simulink model "gm_sampleModel1941_sub"  (R2023a)
settings: Solver=VariableStepAuto  StartTime=0.0  StopTime=10.0  RelTol=1e-3
libraries: simulink x1, hdlsllib x1
settings Model: Creator=user1  LastModifiedBy=user1
settings OptimizationCC: BlockReduction=off  ConditionallyExecuteInputs=off
settings DebuggingCC: InheritedTsInSrcMsg=none

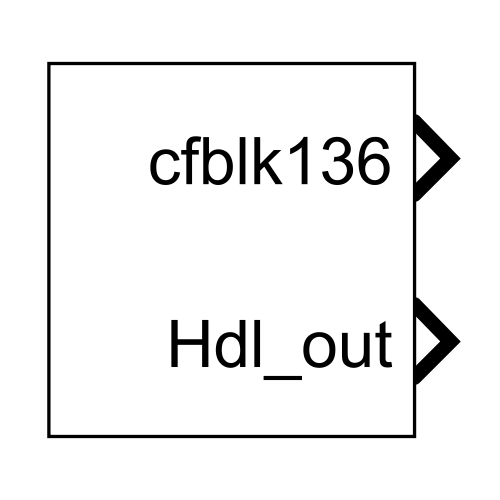
[thumbnail: Simulink's stored preview of the top-level diagram]
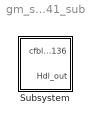
== system gm_sampleModel1941_sub ==
  Subsystem : Subsystem

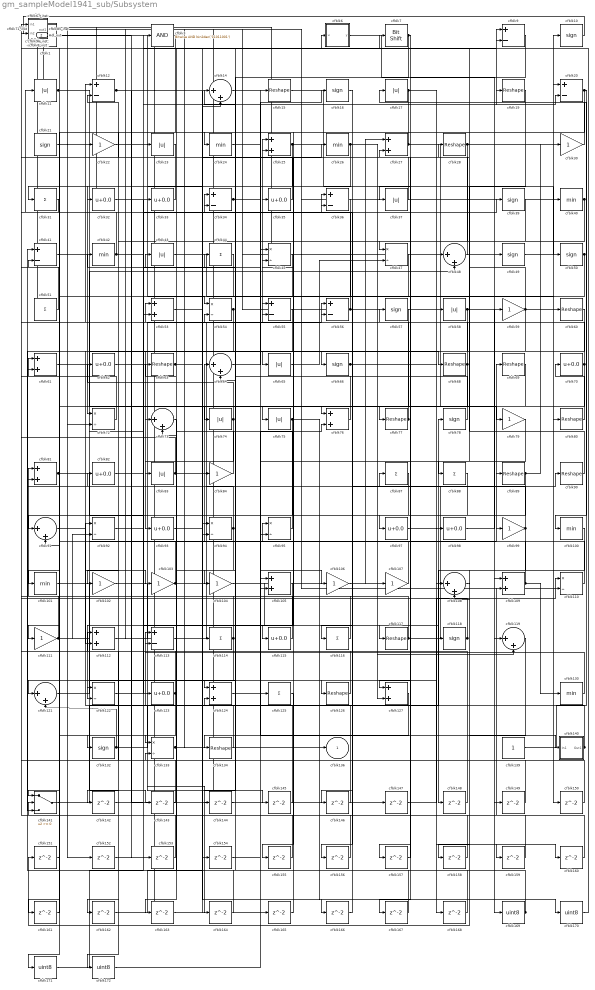
== system gm_sampleModel1941_sub/Subsystem ==
  cfblk1 : Subsystem  mask(Detect Rise Nonnegative){vinit=double(0), InputProcessing=Elements as channels (sample based), OutDataTypeStr=uint8}
      mask prompts: vinit "Simulink:masks:InitialCondition_MP"; InputProcessing "Simulink:masks:InputProcessing_MP"; OutDataTypeStr "Simulink:masks:OutputDataType_MP"
      mask help: Simulink:masks:DetectRiseNonnegative_MD
      mask init:
      | InputProcessing = 'Elements as channels (sample based)';
      | OutDataTypeStr = 'uint8';
      | vinit = double(0);
      mask TypeOptions InputProcessing: Simulink:masks:ColumnsAsChannelsFrameBased | Simulink:masks:ElementsAsChannelsSampleBased
      mask TypeOptions OutDataTypeStr: Simulink:masks:uint8 | Simulink:masks:boolean
      mask Display: fprintf('U >= 0\n&  NOT\nU/z >= 0')
  cfblk{10,16,21,39,49..50,57,66,78,118,132} (11 alike) : Signum
  cfblk{24,26,40,42,100..101,130} (7 alike) : MinMax  OutDataTypeStr=uint8
  cfblk{22,30,59,79,84,99,102..104,106..107,111} (12 alike) : Gain  OutDataTypeStr=uint8
  cfblk{25,27,53,61,76,81,105,109,112,124,127} (11 alike) : Sum  OutDataTypeStr=uint8
  cfblk{14,48,64,73,91,108,119,121} (8 alike) : Sum  Inputs=|++  OutDataTypeStr=uint8
  cfblk{11,17,23,37,43,58,65,74..75,83} (10 alike) : Abs  OutDataTypeStr=uint8  SaturateOnIntegerOverflow=off
  cfblk{45,47,54,72,92,94..95,110,122,133} (10 alike) : Product  Inputs=*/  OutDataTypeStr=uint8  RndMeth=Zero  SaturateOnIntegerOverflow=on
  cfblk{9,12,20,34,36,41,55..56,113} (9 alike) : Sum  Inputs=+-  OutDataTypeStr=uint8
  cfblk{31,44,51,87..88,114,116,125} (8 alike) : Sum  Inputs=+  OutDataTypeStr=uint8
  cfblk{32..33,35,62,70,82,93,97..98,115,123} (11 alike) : Bias  Bias=0.0  SaturateOnIntegerOverflow=off
  cfblk{15,19,28,60,63,68..69,77,80,89..90,117,126,134} (14 alike) : Reshape
  cfblk120_inst : Subsystem
  cfblk128_inst : Subsystem
  cfblk129_inst : Subsystem
  cfblk139 : Constant  OutDataTypeStr=uint8  SampleTime=-1
  cfblk13_inst : Subsystem
  cfblk140 : Subsystem
  cfblk141 : Switch  OutDataTypeStr=uint8  SaturateOnIntegerOverflow=off  InputSameDT=off
  cfblk{142..168} (27 alike) : Delay  SampleTime=1
  cfblk{169..172} (4 alike) : DataTypeConversion  OutDataTypeStr=uint8  SaturateOnIntegerOverflow=off  RndMeth=Floor
  cfblk18_inst : Subsystem
  cfblk2 : Constant  Value=0  OutDataTypeStr=uint8  SampleTime=1
  cfblk29_inst : Subsystem
  cfblk3 : simulink/Logic and Bit Operations/Bitwise Operator  logicop=AND  UseBitMask=on  BitMask=bin2dec('11011001')  BitMaskRealWorld=Stored Integer
      settings: LibrarySourceBlock=|
      | hdlsllib/Logic and Bit
      | Operations/Bitwise
      | Operator
  cfblk4 : Constant  Value=0  OutDataTypeStr=uint8  SampleTime=1
  cfblk46_inst : Subsystem
  cfblk5 : Constant  Value=0  OutDataTypeStr=uint8  SampleTime=1
  cfblk6 : Subsystem  mask(Compare To Constant){relop=<=, const=double(3), OutDataTypeStr=uint8, ZeroCross=on}
      mask prompts: relop "Simulink:masks:Operator_MP"; const "Simulink:masks:ConstantValue_MP"; OutDataTypeStr "Simulink:masks:OutputDataType_MP"; ZeroCross "Simulink:masks:EnableZerocrossingDetection_MP"
      mask help: Simulink:masks:CompareToConstant_MD
      mask init:
      | OutDataTypeStr = 'uint8';
      | ZeroCross = 'on';
      | blkName = 'sampleModel1941_sub/Subsystem/cfblk6';
      | const = double(3);
      | const_str = '3.0';
      | const_val = double(3);
      | relop = '<=';
      | setValue = 'fixdt(0, 8)';
      | str = '<= 3';
      mask TypeOptions relop: == | ~= | < | <= | >= | >
      mask TypeOptions OutDataTypeStr: Simulink:masks:uint8 | Simulink:masks:boolean
      mask Callback ZeroCross: sl('zeroCrossEnable', gcbh);
      mask Display: disp(str)
  cfblk67_inst : Subsystem
  cfblk7 : hdlsllib/Logic and Bit Operations/Bit Shift  mode=Shift Left Logical  N=0
  cfblk71_inst : Subsystem
  cfblk85_inst : Subsystem
  cfblk8_inst : Subsystem
  cfblk96_inst : Subsystem
  cfblk136 : Outport  OutDataTypeStr=uint8  SampleTime=1  VectorParamsAs1DForOutWhenUnconnected=off
  Hdl_out : Outport  Port=2  OutDataTypeStr=uint8  SampleTime=1
  wires:
  cfblk1/1(Y) -> cfblk54/1
  cfblk10/1 -> cfblk128_inst/2(in2)
  cfblk100/1 -> cfblk148/1
  cfblk101/1 -> cfblk143/1
  cfblk102/1 -> cfblk164/1
  cfblk103/1 -> cfblk41/2, cfblk25/1
  cfblk104/1 -> cfblk117/1
  cfblk105/1 -> cfblk122/2
  cfblk106/1 -> cfblk27/1
  cfblk107/1 -> cfblk46_inst/2(in2)
  cfblk108/1 -> cfblk151/1
  cfblk109/1 -> cfblk69/1, cfblk130/1
  cfblk11/1 -> cfblk75/1, Hdl_out/1
  cfblk110/1 -> cfblk35/1
  cfblk111/1 -> cfblk67_inst/2(in2), cfblk48/2, cfblk92/2, cfblk168/1
  cfblk112/1 -> cfblk56/1
  cfblk113/1 -> cfblk89/1
  cfblk114/1 -> cfblk8_inst/2(in2), cfblk121/1
  cfblk115/1 -> cfblk81/1
  cfblk116/1 -> cfblk61/1
  cfblk117/1 -> cfblk90/1, cfblk55/1
  cfblk118/1 -> cfblk71_inst/1(in1), cfblk120_inst/1(in1)
  cfblk119/1 -> cfblk158/1
  cfblk12/1 -> cfblk154/1, cfblk153/1
  cfblk120_inst/1(out1) -> cfblk21/1, cfblk107/1
  cfblk121/1 -> cfblk64/1
  cfblk122/1 -> cfblk145/1
  cfblk123/1 -> cfblk67_inst/1(in1), cfblk161/1
  cfblk124/1 -> cfblk125/1
  cfblk125/1 -> cfblk155/1
  cfblk126/1 -> cfblk46_inst/1(in1)
  cfblk127/1 -> cfblk134/1
  cfblk128_inst/1(out1) -> cfblk15/1
  cfblk129_inst/1(out1) -> cfblk96_inst/2(in2), cfblk152/1, cfblk136/1
  cfblk13_inst/1(out1) -> cfblk50/1
  cfblk130/1 -> cfblk113/1
  cfblk132/1 -> cfblk124/2, cfblk121/2
  cfblk133/1 -> cfblk99/1, cfblk166/1
  cfblk134/1 -> cfblk113/2
  cfblk139/1 -> cfblk17/1
  cfblk14/1 -> cfblk140/1(In1)
  cfblk140/1(Out1) -> cfblk53/1, cfblk87/1
  cfblk141/1 -> cfblk78/1
  cfblk142/1 -> cfblk36/1
  cfblk143/1 -> cfblk18_inst/1(in1)
  cfblk144/1 -> cfblk1/1(U)
  cfblk145/1 -> cfblk92/1
  cfblk146/1 -> cfblk73/2
  cfblk147/1 -> cfblk110/1
  cfblk148/1 -> cfblk61/2
  cfblk149/1 -> cfblk55/2
  cfblk15/1 -> cfblk80/1
  cfblk150/1 -> cfblk112/1
  cfblk151/1 -> cfblk91/2
  cfblk152/1 -> cfblk95/1
  cfblk153/1 -> cfblk96_inst/1(in1)
  cfblk154/1 -> cfblk76/2
  cfblk155/1 -> cfblk29_inst/2(in2)
  cfblk156/1 -> cfblk14/1
  cfblk157/1 -> cfblk27/2
  cfblk158/1 -> cfblk13_inst/1(in1)
  cfblk159/1 -> cfblk109/2
  cfblk16/1 -> cfblk146/1
  cfblk160/1 -> cfblk34/1
  cfblk161/1 -> cfblk141/2
  cfblk162/1 -> cfblk94/1
  cfblk163/1 -> cfblk20/2
  cfblk164/1 -> cfblk133/2
  cfblk165/1 -> cfblk45/2
  cfblk166/1 -> cfblk56/2
  cfblk167/1 -> cfblk25/2
  cfblk168/1 -> cfblk54/2
  cfblk169/1 -> cfblk43/1, cfblk41/1
  cfblk17/1 -> cfblk98/1, cfblk115/1
  cfblk170/1 -> cfblk6/1(u)
  cfblk171/1 -> cfblk3/1
  cfblk172/1 -> cfblk105/1
  cfblk18_inst/1(out1) -> cfblk72/2, cfblk165/1
  cfblk19/1 -> cfblk88/1
  cfblk2/1 -> cfblk33/1
  cfblk20/1 -> cfblk100/1, cfblk31/1
  cfblk21/1 -> cfblk66/1
  cfblk22/1 -> cfblk84/1
  cfblk23/1 -> cfblk72/1
  cfblk24/1 -> cfblk79/1
  cfblk25/1 -> cfblk119/1, cfblk111/1
  cfblk26/1 -> cfblk65/1, cfblk119/2
  cfblk27/1 -> cfblk109/1, cfblk24/1
  cfblk28/1 -> cfblk10/1, cfblk167/1
  cfblk29_inst/1(out1) -> cfblk60/1, cfblk23/1, cfblk110/2
  cfblk3/1 -> cfblk172/1
  cfblk30/1 -> cfblk9/1
  cfblk31/1 -> cfblk11/1
  cfblk32/1 -> cfblk118/1
  cfblk33/1 -> cfblk32/1
  cfblk34/1 -> cfblk124/1, cfblk106/1
  cfblk35/1 -> cfblk18_inst/2(in2)
  cfblk36/1 -> cfblk53/2
  cfblk37/1 -> cfblk129_inst/1(in1)
  cfblk39/1 -> cfblk132/1
  cfblk4/1 -> cfblk22/1
  cfblk40/1 -> cfblk74/1, cfblk95/2
  cfblk41/1 -> cfblk149/1
  cfblk42/1 -> cfblk71_inst/2(in2), cfblk19/1
  cfblk43/1 -> cfblk150/1
  cfblk44/1 -> cfblk162/1
  cfblk45/1 -> cfblk104/1
  cfblk46_inst/1(out1) -> cfblk58/1
  cfblk47/1 -> cfblk144/1
  cfblk48/1 -> cfblk12/2
  cfblk49/1 -> cfblk20/1
  cfblk5/1 -> cfblk49/1
  cfblk50/1 -> cfblk76/1, cfblk171/1
  cfblk51/1 -> cfblk8_inst/1(in1)
  cfblk53/1 -> cfblk39/1
  cfblk54/1 -> cfblk91/1, cfblk141/3
  cfblk55/1 -> cfblk112/2
  cfblk56/1 -> cfblk85_inst/2(in2), cfblk116/1
  cfblk57/1 -> cfblk122/1
  cfblk58/1 -> cfblk97/1, cfblk93/1
  cfblk59/1 -> cfblk129_inst/2(in2), cfblk127/1
  cfblk6/1(y) -> cfblk169/1
  cfblk60/1 -> cfblk127/2
  cfblk61/1 -> cfblk73/1
  cfblk62/1 -> cfblk68/1
  cfblk63/1 -> cfblk14/2, cfblk126/1
  cfblk64/1 -> cfblk16/1
  cfblk65/1 -> cfblk47/2
  cfblk66/1 -> cfblk160/1, cfblk159/1
  cfblk67_inst/1(out1) -> cfblk40/1
  cfblk68/1 -> cfblk77/1, cfblk57/1, cfblk157/1
  cfblk69/1 -> cfblk101/1
  cfblk7/1 -> cfblk64/2, cfblk37/1
  cfblk70/1 -> cfblk34/2, cfblk142/1
  cfblk71_inst/1(out1) -> cfblk114/1
  cfblk72/1 -> cfblk128_inst/1(in1)
  cfblk73/1 -> cfblk133/1
  cfblk74/1 -> cfblk83/1, cfblk62/1
  cfblk75/1 -> cfblk170/1, cfblk94/2
  cfblk76/1 -> cfblk42/1
  cfblk77/1 -> cfblk85_inst/1(in1), cfblk12/1
  cfblk78/1 -> cfblk13_inst/2(in2)
  cfblk79/1 -> cfblk105/2
  cfblk8_inst/1(out1) -> cfblk147/1
  cfblk80/1 -> cfblk70/1
  cfblk81/1 -> cfblk123/1, cfblk44/1
  cfblk82/1 -> cfblk9/2
  cfblk83/1 -> cfblk120_inst/2(in2), cfblk26/1
  cfblk84/1 -> cfblk29_inst/1(in1)
  cfblk85_inst/1(out1) -> cfblk51/1
  cfblk87/1 -> cfblk156/1
  cfblk88/1 -> cfblk102/1
  cfblk89/1 -> cfblk141/1, cfblk30/1
  cfblk9/1 -> cfblk47/1
  cfblk90/1 -> cfblk28/1
  cfblk91/1 -> cfblk103/1
  cfblk92/1 -> cfblk45/1
  cfblk93/1 -> cfblk7/1
  cfblk94/1 -> cfblk82/1, cfblk81/2, cfblk163/1
  cfblk95/1 -> cfblk63/1
  cfblk96_inst/1(out1) -> cfblk48/1
  cfblk97/1 -> cfblk108/1
  cfblk98/1 -> cfblk59/1
  cfblk99/1 -> cfblk36/2, cfblk108/2

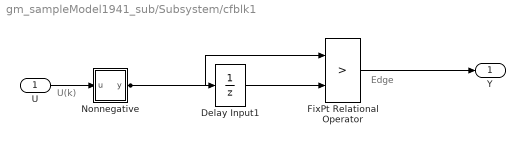
== system gm_sampleModel1941_sub/Subsystem/cfblk1 ==
  note: U(k)
  note: Edge
  U : Inport  OutDataTypeStr=uint8  SampleTime=1
  Delay Input1 : UnitDelay  Description=Store in Global RAM  DisableCoverage=on  InitialCondition=vinit  SampleTime=-1  HasFrameUpgradeWarning=on
  FixPt Relational Operator : RelationalOperator  Operator=>  OutDataTypeStr=fixdt(0, 8)  ZeroCross=off  InputSameDT=off
  Nonnegative : Subsystem  mask(Compare To Zero){relop=>=, OutDataTypeStr=boolean, ZeroCross=off}
      mask prompts: relop "Simulink:masks:Operator_MP"; OutDataTypeStr "Simulink:masks:OutputDataType_MP"; ZeroCross "Simulink:masks:EnableZerocrossingDetection_MP"
      mask help: Simulink:masks:CompareToZero_MD
      mask init:
      | OutDataTypeStr = 'boolean';
      | ZeroCross = 'off';
      | blkName = 'sampleModel1941_sub/Subsystem/cfblk1/Nonnegative';
      | relop = '>=';
      | setValue = 'boolean';
      mask TypeOptions relop: == | ~= | < | <= | >= | >
      mask TypeOptions OutDataTypeStr: Simulink:masks:uint8 | Simulink:masks:boolean
      mask Callback ZeroCross: sl('zeroCrossEnable', gcbh);
      mask Display: disp([relop,' 0'])
  Y : Outport  SampleTime=1
  wires:
  U/1 -> Nonnegative/1(u)
  Delay Input1/1 -> FixPt Relational Operator/2
  FixPt Relational Operator/1 -> Y/1
  Nonnegative/1(y) -> FixPt Relational Operator/1, Delay Input1/1

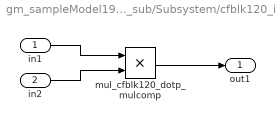
== system gm_sampleModel1941_sub/Subsystem/cfblk120_inst ==
  in1 : Inport  OutDataTypeStr=uint8  SampleTime=1
  in2 : Inport  Port=2  OutDataTypeStr=uint8  SampleTime=1
  mul_cfblk120_dotp_mulcomp : Product  Inputs=**  OutDataTypeStr=uint8  SampleTime=1
  out1 : Outport  OutDataTypeStr=uint8  SampleTime=1
  wires:
  in1/1 -> mul_cfblk120_dotp_mulcomp/1
  in2/1 -> mul_cfblk120_dotp_mulcomp/2
  mul_cfblk120_dotp_mulcomp/1 -> out1/1

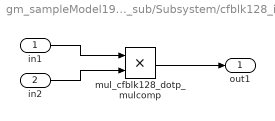
== system gm_sampleModel1941_sub/Subsystem/cfblk128_inst ==
  in1 : Inport  OutDataTypeStr=uint8  SampleTime=1
  in2 : Inport  Port=2  OutDataTypeStr=uint8  SampleTime=1
  mul_cfblk128_dotp_mulcomp : Product  Inputs=**  OutDataTypeStr=uint8  SampleTime=1
  out1 : Outport  OutDataTypeStr=uint8  SampleTime=1
  wires:
  in1/1 -> mul_cfblk128_dotp_mulcomp/1
  in2/1 -> mul_cfblk128_dotp_mulcomp/2
  mul_cfblk128_dotp_mulcomp/1 -> out1/1

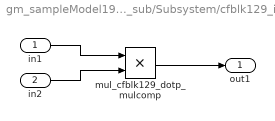
== system gm_sampleModel1941_sub/Subsystem/cfblk129_inst ==
  in1 : Inport  OutDataTypeStr=uint8  SampleTime=1
  in2 : Inport  Port=2  OutDataTypeStr=uint8  SampleTime=1
  mul_cfblk129_dotp_mulcomp : Product  Inputs=**  OutDataTypeStr=uint8  SampleTime=1
  out1 : Outport  OutDataTypeStr=uint8  SampleTime=1
  wires:
  in1/1 -> mul_cfblk129_dotp_mulcomp/1
  in2/1 -> mul_cfblk129_dotp_mulcomp/2
  mul_cfblk129_dotp_mulcomp/1 -> out1/1

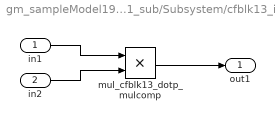
== system gm_sampleModel1941_sub/Subsystem/cfblk13_inst ==
  in1 : Inport  OutDataTypeStr=uint8  SampleTime=1
  in2 : Inport  Port=2  OutDataTypeStr=uint8  SampleTime=1
  mul_cfblk13_dotp_mulcomp : Product  Inputs=**  OutDataTypeStr=uint8  SampleTime=1
  out1 : Outport  OutDataTypeStr=uint8  SampleTime=1
  wires:
  in1/1 -> mul_cfblk13_dotp_mulcomp/1
  in2/1 -> mul_cfblk13_dotp_mulcomp/2
  mul_cfblk13_dotp_mulcomp/1 -> out1/1

== system gm_sampleModel1941_sub/Subsystem/cfblk140 ==
  In1 : Inport  OutDataTypeStr=uint8  PortDimensions=1  SampleTime=1
  Out1 : Outport  SampleTime=1
  wires:
  In1/1 -> Out1/1

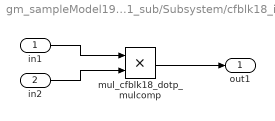
== system gm_sampleModel1941_sub/Subsystem/cfblk18_inst ==
  in1 : Inport  OutDataTypeStr=uint8  SampleTime=1
  in2 : Inport  Port=2  OutDataTypeStr=uint8  SampleTime=1
  mul_cfblk18_dotp_mulcomp : Product  Inputs=**  OutDataTypeStr=uint8  SampleTime=1
  out1 : Outport  OutDataTypeStr=uint8  SampleTime=1
  wires:
  in1/1 -> mul_cfblk18_dotp_mulcomp/1
  in2/1 -> mul_cfblk18_dotp_mulcomp/2
  mul_cfblk18_dotp_mulcomp/1 -> out1/1

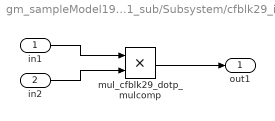
== system gm_sampleModel1941_sub/Subsystem/cfblk29_inst ==
  in1 : Inport  OutDataTypeStr=uint8  SampleTime=1
  in2 : Inport  Port=2  OutDataTypeStr=uint8  SampleTime=1
  mul_cfblk29_dotp_mulcomp : Product  Inputs=**  OutDataTypeStr=uint8  SampleTime=1
  out1 : Outport  OutDataTypeStr=uint8  SampleTime=1
  wires:
  in1/1 -> mul_cfblk29_dotp_mulcomp/1
  in2/1 -> mul_cfblk29_dotp_mulcomp/2
  mul_cfblk29_dotp_mulcomp/1 -> out1/1

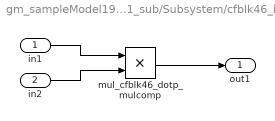
== system gm_sampleModel1941_sub/Subsystem/cfblk46_inst ==
  in1 : Inport  OutDataTypeStr=uint8  SampleTime=1
  in2 : Inport  Port=2  OutDataTypeStr=uint8  SampleTime=1
  mul_cfblk46_dotp_mulcomp : Product  Inputs=**  OutDataTypeStr=uint8  SampleTime=1
  out1 : Outport  OutDataTypeStr=uint8  SampleTime=1
  wires:
  in1/1 -> mul_cfblk46_dotp_mulcomp/1
  in2/1 -> mul_cfblk46_dotp_mulcomp/2
  mul_cfblk46_dotp_mulcomp/1 -> out1/1

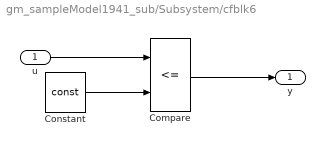
== system gm_sampleModel1941_sub/Subsystem/cfblk6 ==
  u : Inport  OutDataTypeStr=uint8  SampleTime=1
  Compare : RelationalOperator  Operator=<=  OutDataTypeStr=fixdt(0, 8)
  Constant : Constant  DisableCoverage=on  Value=const  OutDataTypeStr=Inherit: Inherit via back propagation  SampleTime=-1
  y : Outport  SampleTime=1
  wires:
  u/1 -> Compare/1
  Compare/1 -> y/1
  Constant/1 -> Compare/2

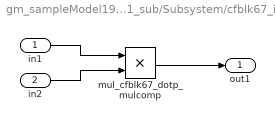
== system gm_sampleModel1941_sub/Subsystem/cfblk67_inst ==
  in1 : Inport  OutDataTypeStr=uint8  SampleTime=1
  in2 : Inport  Port=2  OutDataTypeStr=uint8  SampleTime=1
  mul_cfblk67_dotp_mulcomp : Product  Inputs=**  OutDataTypeStr=uint8  SampleTime=1
  out1 : Outport  OutDataTypeStr=uint8  SampleTime=1
  wires:
  in1/1 -> mul_cfblk67_dotp_mulcomp/1
  in2/1 -> mul_cfblk67_dotp_mulcomp/2
  mul_cfblk67_dotp_mulcomp/1 -> out1/1

== system gm_sampleModel1941_sub/Subsystem/cfblk71_inst ==
  in1 : Inport  OutDataTypeStr=uint8  SampleTime=1
  in2 : Inport  Port=2  OutDataTypeStr=uint8  SampleTime=1
  mul_cfblk71_dotp_mulcomp : Product  Inputs=**  OutDataTypeStr=uint8  SampleTime=1
  out1 : Outport  OutDataTypeStr=uint8  SampleTime=1
  wires:
  in1/1 -> mul_cfblk71_dotp_mulcomp/1
  in2/1 -> mul_cfblk71_dotp_mulcomp/2
  mul_cfblk71_dotp_mulcomp/1 -> out1/1

== system gm_sampleModel1941_sub/Subsystem/cfblk85_inst ==
  in1 : Inport  OutDataTypeStr=uint8  SampleTime=1
  in2 : Inport  Port=2  OutDataTypeStr=uint8  SampleTime=1
  mul_cfblk85_dotp_mulcomp : Product  Inputs=**  OutDataTypeStr=uint8  SampleTime=1
  out1 : Outport  OutDataTypeStr=uint8  SampleTime=1
  wires:
  in1/1 -> mul_cfblk85_dotp_mulcomp/1
  in2/1 -> mul_cfblk85_dotp_mulcomp/2
  mul_cfblk85_dotp_mulcomp/1 -> out1/1

== system gm_sampleModel1941_sub/Subsystem/cfblk8_inst ==
  in1 : Inport  OutDataTypeStr=uint8  SampleTime=1
  in2 : Inport  Port=2  OutDataTypeStr=uint8  SampleTime=1
  mul_cfblk8_dotp_mulcomp : Product  Inputs=**  OutDataTypeStr=uint8  SampleTime=1
  out1 : Outport  OutDataTypeStr=uint8  SampleTime=1
  wires:
  in1/1 -> mul_cfblk8_dotp_mulcomp/1
  in2/1 -> mul_cfblk8_dotp_mulcomp/2
  mul_cfblk8_dotp_mulcomp/1 -> out1/1

== system gm_sampleModel1941_sub/Subsystem/cfblk96_inst ==
  in1 : Inport  OutDataTypeStr=uint8  SampleTime=1
  in2 : Inport  Port=2  OutDataTypeStr=uint8  SampleTime=1
  mul_cfblk96_dotp_mulcomp : Product  Inputs=**  OutDataTypeStr=uint8  SampleTime=1
  out1 : Outport  OutDataTypeStr=uint8  SampleTime=1
  wires:
  in1/1 -> mul_cfblk96_dotp_mulcomp/1
  in2/1 -> mul_cfblk96_dotp_mulcomp/2
  mul_cfblk96_dotp_mulcomp/1 -> out1/1

== system gm_sampleModel1941_sub/Subsystem/cfblk1/Nonnegative ==
  u : Inport  OutDataTypeStr=uint8  SampleTime=1
  Compare : RelationalOperator  OutDataTypeStr=boolean  ZeroCross=off
  Constant : Constant  DisableCoverage=on  Value=0  OutDataTypeStr=Inherit: Inherit via back propagation  SampleTime=-1  PreserveConstantTs=on
  y : Outport  SampleTime=1
  wires:
  u/1 -> Compare/1
  Compare/1 -> y/1
  Constant/1 -> Compare/2
